simulink model "PX50"  (R2015b)
settings: Solver=VariableStepAuto  StartTime=0.0  StopTime=3  RelTol=1e-3
settings Model: Creator=xmax1946  LastModifiedBy=xmax1946

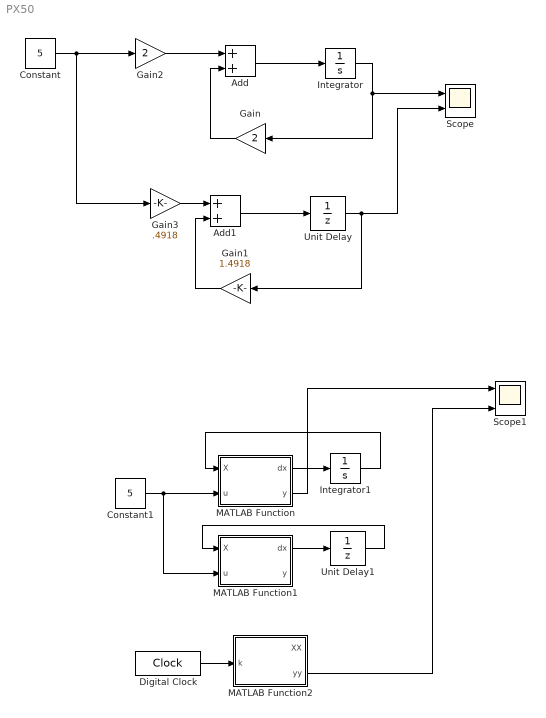
== system PX50 ==
  Add : Sum
  Add1 : Sum
  Constant : Constant  Value=5
  Constant1 : Constant  Value=5
  Digital Clock : DigitalClock
  Gain : Gain  Gain=2
  Gain1 : Gain  Gain=1.4918
  Gain2 : Gain  Gain=2
  Gain3 : Gain  Gain=.4918
  Integrator : Integrator  InitialCondition=-1
  Integrator1 : Integrator  InitialCondition=[-1,-1]
  MATLAB Function : MATLAB Function  TreatAsAtomicUnit=on
  MATLAB Function1 : MATLAB Function  TreatAsAtomicUnit=on
  MATLAB Function2 : MATLAB Function  TreatAsAtomicUnit=on
  Scope : Scope  NumInputPorts=2
  Scope1 : Scope  NumInputPorts=3
  Unit Delay : UnitDelay  InitialCondition=-1  SampleTime=.2
  Unit Delay1 : UnitDelay  InitialCondition=[-1,-1]  SampleTime=.2
  wires:
  Integrator/1 -> Scope/1, Gain/1
  Add/1 -> Integrator/1
  Gain/1 -> Add/2
  Add1/1 -> Unit Delay/1
  Gain1/1 -> Add1/2
  Gain2/1 -> Add/1
  Gain3/1 -> Add1/1
  Unit Delay/1 -> Gain1/1, Scope/2
  Constant/1 -> Gain3/1, Gain2/1
  MATLAB Function/1(dx) -> Integrator1/1
  Integrator1/1 -> MATLAB Function/1(X)
  Constant1/1 -> MATLAB Function1/2(u), MATLAB Function/2(u)
  MATLAB Function1/1(dx) -> Unit Delay1/1
  Unit Delay1/1 -> MATLAB Function1/1(X)
  MATLAB Function/2(y) -> Scope1/1
  MATLAB Function2/2(yy) -> Scope1/3
  Digital Clock/1 -> MATLAB Function2/1(k)

== matlab function PX50/MATLAB Function1 ==
  data: X input; dx output; u input; y output
function [dx,y] = fcn(X,u)

A=[1.4918246976412703178248529528372, 0.13263076110394170116926744414386
   0,1.173510870991810235018611086892];
B=[-1.2053752773691154902794968672567
 0.43377717747952558754652771722991];
C=[1,1];

dx=A*X+B*u;
y=C*X;

== matlab function PX50/MATLAB Function ==
  data: X input; dx output; u input; y output
function [dx,y] = fcn(X,u)

A=[2,.5;0,.8];
B=[-5;2];
C=[1,1];

dx=A*X+B*u;
y=C*X;

== matlab function PX50/MATLAB Function2 ==
  data: k input; XX output; yy output
function [XX,yy] = fcn(k)
XX=[(85*(4/5)^k)/4 - (89*2^k)/4
             50 - 51*(4/5)^k];
Cc=[1,1];
yy=Cc*XX;
